simulink model "simcape_real_time_V3"  (R2022b)
settings: Solver=FixedStepAuto  StartTime=0.0  StopTime=100  FixedStep=0.002  RelTol=1e-3
undefined symbols (not defined in the file): drone_leg, K_LQR_GOC, pitch_init, roll_init, v_pitch_init, v_roll_init, v_x_init, v_y_init, v_yaw_init, v_z_init, X, x_init, Y, y_init, yaw_init, Z, z_init
libraries: sm_lib x70, nesl_utility x11, simulink x6
(part 1 of 4)
settings Model: Creator=tridu  LastModifiedBy=tridu

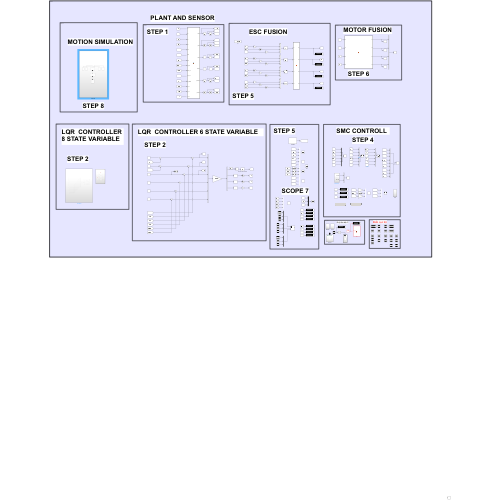
[thumbnail: Simulink's stored preview of the top-level diagram]
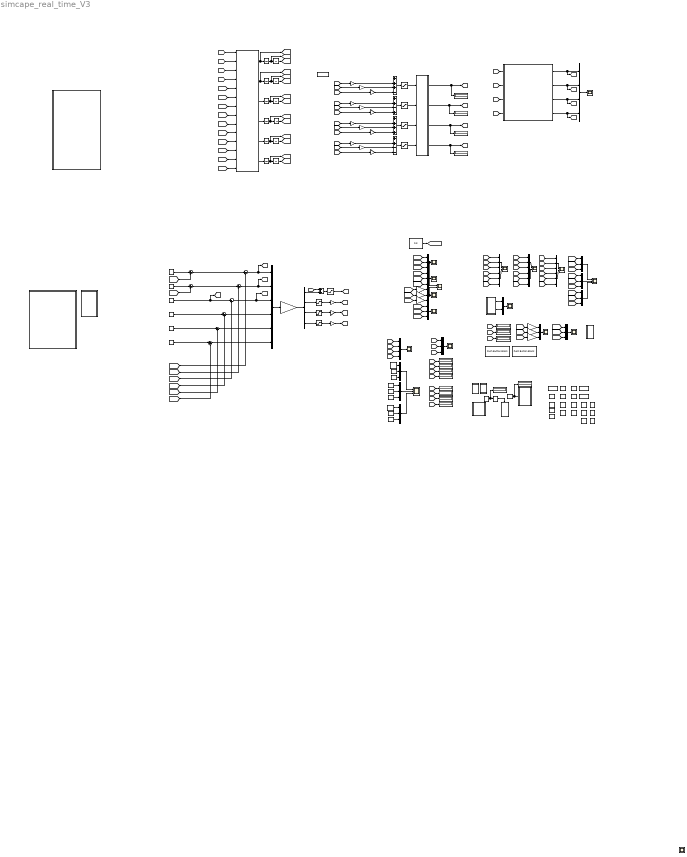
== system simcape_real_time_V3 ==
  note: STEP 2
  note: Quỹ đạo bậc 5
  note: LQR CONTROLLER 8 STATE VARIABLE
  note: Biến cục bộ
  note: Quỹ đạo
  note: STEP 5
  note: ARM 2
  note: ARM 2
  note: STEP 4
  note: ARM 2
  note: STEP 1
  note: SCOPE 7
  note: STEP 6
  note: ARM 2
  note: STEP 5
  note: SMC CONTROLL
  note: PLANT AND SENSOR
  note: LQR CONTROLLER 6 STATE VARIABLE
  note: ARM 2
  note: STEP 8
  note: MOTOR FUSION
  note: ARM 2
  note: ARM 2
  note: ARM 2
  note: ESC FUSION
  note: STEP 2
  note: MOTION SIMULATION
  Add : Sum
  Add1 : Sum  Inputs=+++-
  Add3 : Sum  Inputs=++-+
  Add4 : Sum  Inputs=++++
  Add5 : Sum  Inputs=++--
  Compare To Constant : simulink/Logic and Bit Operations/Compare To Constant  relop===  const=1  OutDataTypeStr=boolean
  Constant : Constant  Value=1.7*9.81/4
  Constant{2..3,23,25..27} (6 alike) : Constant  Value=0
  Data Store Memory : DataStoreMemory  DataStoreName=x_a  WriteAfterWriteMsg=warning  ShowAdditionalParam=off
  Data Store Memory1 : DataStoreMemory  DataStoreName=z_a  WriteAfterWriteMsg=warning  ShowAdditionalParam=off
  Data Store Memory10 : DataStoreMemory  DataStoreName=start  WriteAfterWriteMsg=warning  ShowAdditionalParam=off
  Data Store Memory11 : DataStoreMemory  DataStoreName=v_x  WriteAfterWriteMsg=warning  ShowAdditionalParam=off
  Data Store Memory12 : DataStoreMemory  DataStoreName=v_y  WriteAfterWriteMsg=warning  ShowAdditionalParam=off
  Data Store Memory13 : DataStoreMemory  DataStoreName=enable  WriteAfterWriteMsg=warning  ShowAdditionalParam=off
  Data Store Memory14 : DataStoreMemory  DataStoreName=stop  WriteAfterWriteMsg=warning  ShowAdditionalParam=off
  Data Store Memory15 : DataStoreMemory  DataStoreName=motor_13  WriteAfterWriteMsg=warning  ShowAdditionalParam=off  OutDataTypeStr=double  Dimensions=1
  Data Store Memory16 : DataStoreMemory  DataStoreName=motor_24  WriteAfterWriteMsg=warning  ShowAdditionalParam=off  OutDataTypeStr=double  Dimensions=1
  Data Store Memory17 : DataStoreMemory  DataStoreName=v_z  WriteAfterWriteMsg=warning  ShowAdditionalParam=off
  Data Store Memory18 : DataStoreMemory  DataStoreName=a_x  WriteAfterWriteMsg=warning  ShowAdditionalParam=off
  Data Store Memory19 : DataStoreMemory  DataStoreName=a_y  WriteAfterWriteMsg=warning  ShowAdditionalParam=off
  Data Store Memory2 : DataStoreMemory  DataStoreName=y_a  WriteAfterWriteMsg=warning  ShowAdditionalParam=off
  Data Store Memory20 : DataStoreMemory  DataStoreName=a_z  WriteAfterWriteMsg=warning  ShowAdditionalParam=off
  Data Store Memory3 : DataStoreMemory  DataStoreName=t  WriteAfterWriteMsg=warning  ShowAdditionalParam=off
  Data Store Memory4 : DataStoreMemory  DataStoreName=xyzv  WriteAfterWriteMsg=warning  ShowAdditionalParam=off  OutDataTypeStr=double  Dimensions=4
  Data Store Memory5 : DataStoreMemory  DataStoreName=Px_pre  WriteAfterWriteMsg=warning  ShowAdditionalParam=off
  Data Store Memory6 : DataStoreMemory  DataStoreName=Py_pre  WriteAfterWriteMsg=warning  ShowAdditionalParam=off
  Data Store Memory7 : DataStoreMemory  DataStoreName=Pz_pre  WriteAfterWriteMsg=warning  ShowAdditionalParam=off
  Data Store Memory8 : DataStoreMemory  DataStoreName=phantram_s  WriteAfterWriteMsg=warning  ShowAdditionalParam=off
  Data Store Memory9 : DataStoreMemory  DataStoreName=N_wp  WriteAfterWriteMsg=warning  ShowAdditionalParam=off
  Data Store Read : DataStoreRead  DataStoreName=v_x  IndexOptions=Index vector (dialog)  Indices=1  OutputSizes=1
  Data Store Read14 : DataStoreRead  DataStoreName=a_y  IndexOptions=Index vector (dialog)  Indices=1  OutputSizes=1
  Data Store Read15 : DataStoreRead  DataStoreName=Px_pre  IndexOptions=Index vector (dialog)  Indices=1  OutputSizes=1
  Data Store Read16 : DataStoreRead  DataStoreName=v_z  IndexOptions=Index vector (dialog)  Indices=1  OutputSizes=1
  Data Store Read17 : DataStoreRead  DataStoreName=a_z  IndexOptions=Index vector (dialog)  Indices=1  OutputSizes=1
  Data Store Read2 : DataStoreRead  DataStoreName=N_wp  DataStoreElements=N_wp  IndexOptions=Index vector (dialog)  Indices=1  OutputSizes=1
  Data Store Read3 : DataStoreRead  DataStoreName=Px_pre  IndexOptions=Index vector (dialog)  Indices=1  OutputSizes=1
  Data Store Read4 : DataStoreRead  DataStoreName=a_x  IndexOptions=Index vector (dialog)  Indices=1  OutputSizes=1
  Data Store Read7 : DataStoreRead  DataStoreName=v_y  IndexOptions=Index vector (dialog)  Indices=1  OutputSizes=1
  Data Store Read8 : DataStoreRead  DataStoreName=Pz_pre  IndexOptions=Index vector (dialog)  Indices=1  OutputSizes=1
  Data Store Read9 : DataStoreRead  DataStoreName=enable  IndexOptions=Index vector (dialog)  Indices=1  OutputSizes=1
  Demux2 : Demux
  Display{,1..12,14..17} (17 alike) : Display
  G00(xyzv) : Subsystem  TreatAsAtomicUnit=on
  Gain{8..12,14,16,18} (8 alike) : Gain  Gain=1/4
  Gain{13,15,17,19} (4 alike) : Gain  Gain=1/2
  Gain20 : Gain  Gain=0.3
  Gain24 : Gain  Gain=0.3
  Gain26 : Gain  Gain=0.1
  Gain{4..6,28..30} (6 alike) : Gain  Gain=180/pi
  Gain7 : Gain  Gain=K_LQR_GOC  Multiplication=Matrix(K*u)
  Giới hạn công suất U2 : Saturate  UpperLimit=11.5*4-1.7*9.81  LowerLimit=-1.7*9.81
  HS_MSKK : Constant  Value=0.3
  Integrator : Integrator  InitialCondition=v_x_init
  Integrator1 : Integrator  InitialCondition=x_init
  Integrator10 : Integrator  InitialCondition=v_yaw_init
  Integrator11 : Integrator  InitialCondition=yaw_init
  Integrator2 : Integrator  InitialCondition=v_y_init
  Integrator3 : Integrator  InitialCondition=y_init
  Integrator4 : Integrator  InitialCondition=z_init
  Integrator5 : Integrator  InitialCondition=v_z_init
  Integrator6 : Integrator  InitialCondition=v_roll_init
  Integrator7 : Integrator  InitialCondition=roll_init
  Integrator8 : Integrator  InitialCondition=v_pitch_init
  Integrator9 : Integrator  InitialCondition=pitch_init
  MATLAB Function : MATLAB Function  TreatAsAtomicUnit=on
  MATLAB Function1 : MATLAB Function  TreatAsAtomicUnit=on
  MATLAB Function2 : MATLAB Function  TreatAsAtomicUnit=on
  Mux{,1..3,6..9,13..23} (19 alike) : Mux  Inputs=3
  Mux10 : Mux  Inputs=6
  Mux11 : Mux
  Mux12 : Mux  Inputs=2
  Mux4 : Mux
  Nút Start : Subsystem
  Nút Stop : Subsystem
  Push Button : PushButtonBlock  ButtonText=Start  IconColor=On  OffValue=0.000000
  Push Button1 : PushButtonBlock  ButtonText=Stop  IconColor=On  OffValue=0.000000
  SIMCAPE : Subsystem
  Saturation1 : Saturate  UpperLimit=11.5  LowerLimit=-11.5
  Saturation10 : Saturate  UpperLimit=11.5  LowerLimit=-11.5
  Saturation{2..5} (4 alike) : Saturate  UpperLimit=11.5  LowerLimit=0
  Saturation8 : Saturate  UpperLimit=11.5  LowerLimit=-11.5
  Scope{,1..3,6,11..15,18} (11 alike) : Scope
  Scope16 : Scope  NumInputPorts=2
  Scope17 : Scope  NumInputPorts=3
  Scope20 : Scope  NumInputPorts=2
  Scope4 : Scope  NumInputPorts=3
  Scope9 : Scope  NumInputPorts=2
  State : Scope  NumInputPorts=2
  Subsystem : Subsystem
  Subsystem1 : Subsystem
  Subsystem3 : Subsystem
  Subsystem4 : Subsystem
  Sum : Sum  Inputs=|++
  Sum{1..4,9..10} (6 alike) : Sum  Inputs=|+-
  Sum11 : Sum  Inputs=|++
  call1 : MATLAB Function  TreatAsAtomicUnit=on
  sai số : Subsystem
  tag scope: D1=global, D2=global, D3=global, D4=global, HS_MSKK=global, T1=global, T2=global, T3=global, T4=global, U1=global, U2=global, U3=global, U4=global, e_pitch=global, e_roll=global, e_yaw=global, pitch=global, pitchdot=global, roll=global, rolldot=global, x2dot=global, x=global, xdot=global, y2dot=global, y=global, yaw=global, yaw_SP=global, yawdot=global, ydot=global, z=global, zdot=global
  wires:
  Data Store Read9/1 -> Display12/1, Compare To Constant/1
  [yaw] -> Gain30/1
  Constant27/1 -> Sum/1
  [pitch] -> MATLAB Function/6(pitch)
  Integrator1/1 -> [x]
  [U1] -> Gain12/1
  Mux15/1 -> Scope15/1
  MATLAB Function2/3(D3) -> Display2/1, [D3]
  [z] -> Mux/3
  [U4] -> Display7/1
  [yawdot] -> Mux3/3
  Gain12/1 -> Add5/2
  [pitchdot] -> Mux3/2
  Sum11/1 -> Sum10/1
  [U3] -> Mux11/3
  [U3] -> Display6/1
  [Ux] -> Mux13/1
  MATLAB Function/2(y2dot) -> [y2dot], Integrator2/1
  [pitchdot] -> MATLAB Function/9(pitch_dot)
  MATLAB Function/3(z2dot) -> Integrator4/1
  Gain13/1 -> Add3/4
  Gain11/1 -> Add3/3
  MATLAB Function1/1(T1) -> Mux4/1, [T1]
  Giới hạn công suất U2/1 -> [U1]
  [rolldot] -> Sum2/2
  Saturation3/1 -> MATLAB Function2/2(T2)
  [ydot] -> Mux1/2
  Integrator/1 -> [xdot], Integrator1/1
  Demux2/4 -> Saturation10/1
  HS_MSKK/1 -> [HS_MSKK]
  Gain5/1 -> Mux2/2
  [rolldot] -> MATLAB Function/8(roll_dot)
  Saturation5/1 -> MATLAB Function2/4(T4)
  [U4] -> Gain14/1
  Gain18/1 -> Add5/3
  Gain7/1 -> Demux2/1
  MATLAB Function2/1(D1) -> Display/1, [D1]
  [x] -> Mux/1
  Saturation10/1 -> Gain26/1
  Saturation8/1 -> Gain24/1
  Data Store Read2/1 -> Display11/1, call1/1(N_wp)
  MATLAB Function1/3(T3) -> Mux4/3, [T3]
  MATLAB Function2/4(D4) -> Display3/1, [D4]
  Gain15/1 -> Add1/4
  Integrator3/1 -> [y]
  [U2] -> Display5/1
  [U4] -> Gain18/1
  [roll] -> Gain4/1
  Sum1/1 -> [e_roll], Mux10/1
  [T1] -> MATLAB Function/1(T1)
  [x] -> Mux14/1
  Constant25/1 -> Sum3/1
  Gain29/1 -> Mux15/2
  [U2] -> Gain19/1
  Gain19/1 -> Add5/4
  [roll] -> Gain28/1
  Add4/1 -> Saturation4/1
  MATLAB Function2/2(D2) -> Display1/1, [D2]
  Demux2/2 -> Saturation1/1
  [U4] -> Gain16/1
  Demux2/3 -> Saturation8/1
  Saturation4/1 -> MATLAB Function2/3(T3)
  [U4] -> Gain11/1
  Saturation2/1 -> MATLAB Function2/1(T1)
  Mux4/1 -> Scope6/1
  [D1] -> MATLAB Function1/1(D1)
  Integrator10/1 -> [yawdot], Integrator11/1
  [zdot] -> MATLAB Function/14(z_dot)
  [y] -> Display9/1
  MATLAB Function/1(x2dot) -> [x2dot], Integrator/1
  [T2] -> MATLAB Function/2(T2)
  Gain28/1 -> Mux15/1
  [U3] -> Gain17/1
  Gain14/1 -> Add1/3
  [D2] -> MATLAB Function1/2(D2)
  MATLAB Function1/4(T4) -> Mux4/4, [T4]
  Mux12/1 -> Scope12/1
  [z] -> Display10/1
  Constant2/1 -> Sum11/1
  Add1/1 -> Saturation2/1
  [Uy] -> Mux13/2
  [U2] -> Gain13/1
  [pitch] -> Sum10/2
  Mux/1 -> State/1, Scope/1
  [y] -> Mux/2
  [yawdot] -> MATLAB Function/10(yaw_dot)
  MATLAB Function1/2(T2) -> Mux4/2, [T2]
  Integrator5/1 -> [z]
  Gain16/1 -> Add4/3
  [D4] -> MATLAB Function1/4(D4)
  Saturation1/1 -> Gain20/1
  [xdot] -> Mux1/1
  Constant26/1 -> Sum4/1
  Add3/1 -> Saturation3/1
  Sum3/1 -> Mux10/5
  Integrator2/1 -> [ydot], Integrator3/1
  [U1] -> Gain10/1
  [U2] -> Mux11/2
  Gain9/1 -> Add3/2
  [U4] -> Mux11/4
  Sum/1 -> Sum1/1
  Sum4/1 -> Mux10/6
  Subsystem4/2(Pitch SP) -> Mux12/2
  Gain8/1 -> Add1/2
  Gain4/1 -> Mux2/1
  [U1] -> Gain9/1
  Integrator6/1 -> [rolldot], Integrator7/1
  Constant23/1 -> Sum2/1
  [pitch] -> Gain5/1
  [U1] -> Gain8/1
  Gain17/1 -> Add4/4
  MATLAB Function/5(pitch2dot) -> Integrator8/1
  Sum10/1 -> [e_pitch], Mux10/2
  [U1] -> Mux11/1
  [roll_SP] -> Sum/2
  Mux13/1 -> Scope13/1
  [T1] -> Display14/1
  [xdot] -> MATLAB Function/12(x_dot)
  [x] -> Display8/1
  [T4] -> Display17/1
  [D3] -> MATLAB Function1/3(D3)
  Gain26/1 -> [U4]
  Subsystem4/1(Roll SP) -> Mux12/1
  MATLAB Function/6(yaw2dot) -> Integrator10/1
  Integrator9/1 -> [pitch]
  Integrator11/1 -> [yaw]
  [z] -> Mux14/3
  [ydot] -> MATLAB Function/13(y_dot)
  [roll] -> MATLAB Function/5(roll)
  [roll] -> Sum1/2
  Gain10/1 -> Add4/2
  Mux10/1 -> Gain7/1
  Gain6/1 -> Mux2/3
  Integrator4/1 -> [zdot], Integrator5/1
  Mux11/1 -> Scope11/1
  [rolldot] -> Mux3/1
  [T3] -> MATLAB Function/3(T3)
  Gain30/1 -> Mux15/3
  MATLAB Function/4(roll2dot) -> Integrator6/1
  Mux3/1 -> Scope3/1
  [yaw] -> Sum9/2
  [U3] -> Gain15/1
  Integrator7/1 -> [roll]
  [U1] -> Display4/1
  Mux1/1 -> Scope1/1
  Integrator8/1 -> [pitchdot], Integrator9/1
  Mux2/1 -> State/2, Scope2/1
  [HS_MSKK] -> MATLAB Function/11(HS_MSKK)
  [y] -> Mux14/2
  [yawdot] -> Sum4/2
  Mux14/1 -> Scope14/1
  Gain20/1 -> [U2]
  [T4] -> MATLAB Function/4(T4)
  [pitch_SP] -> Sum11/2
  [yaw] -> Gain6/1
  Add5/1 -> Saturation5/1
  [pitch] -> Gain29/1
  [pitchdot] -> Sum3/2
  [T3] -> Display16/1
  Gain24/1 -> [U3]
  [yaw] -> MATLAB Function/7(yaw)
  [T2] -> Display15/1
  [Uz] -> Mux13/3
  Sum2/1 -> Mux10/4
  [zdot] -> Mux1/3
  Compare To Constant/1 -> Subsystem/Enable
  Mux9/1 -> Scope17/1
  Data Store Read3/1 -> Mux9/1
  Data Store Read/1 -> Mux9/2
  Data Store Read4/1 -> Mux9/3
  Mux16/1 -> Scope17/2
  Data Store Read14/1 -> Mux16/3
  Data Store Read7/1 -> Mux16/2
  Data Store Read15/1 -> Mux16/1
  Data Store Read16/1 -> Mux17/3
  Data Store Read17/1 -> Mux17/2
  Data Store Read8/1 -> Mux17/1
  Mux17/1 -> Scope17/3
  Sum9/1 -> [e_yaw], Mux10/3
  Constant3/1 -> [yaw_SP], Sum9/1
  [roll_SP] -> Mux21/1
  [e_roll] -> Mux21/3
  [roll] -> Mux21/2
  Mux21/1 -> Scope4/1
  [pitch_SP] -> Mux6/1
  [pitch] -> Mux6/2
  [e_pitch] -> Mux6/3
  [e_yaw] -> Mux7/3
  [yaw_SP] -> Mux7/1
  [yaw] -> Mux7/2
  [x] -> Mux8/2
  Mux8/1 -> Scope9/1
  [xdot] -> Mux18/2
  Mux18/1 -> Scope9/2
  Mux19/1 -> Scope16/2
  Mux20/1 -> Scope16/1
  [y] -> Mux20/2
  [ydot] -> Mux19/2
  Mux22/1 -> Scope20/2
  Mux23/1 -> Scope20/1
  Mux6/1 -> Scope4/2
  Mux7/1 -> Scope4/3
  [z] -> Mux23/2
  [z_SP] -> Mux23/1
  [zdot] -> Mux22/2
  [zdot_SP] -> Mux22/1
  [ez] -> Mux23/3
  [ez_dot] -> Mux22/3
  [xdot_SP] -> Mux18/1
  [x_SP] -> Mux8/1
  [y_SP] -> Mux20/1
  [ydot_SP] -> Mux19/1
  [ex] -> Mux8/3
  [ex_dot] -> Mux18/3
  [ey] -> Mux20/3
  [ey_dot] -> Mux19/3
  Add/1 -> Giới hạn công suất U2/1
  [Uz] -> Add/1
  Demux2/1 -> Add/2

== system simcape_real_time_V3/G00(xyzv) ==
  MoveL : TriggerPort  TriggerType=function-call  IsSimulinkFunction=on  FunctionName=MoveL  FunctionVisibility=scoped  VariantControl=(inherit)
  Data Store Write2 : DataStoreWrite  DataStoreName=xyzv  IndexOptions=Index vector (dialog)  Indices=1  OutputSizes=1
  Display : Display
  Display1 : Display
  MATLAB Function1 : MATLAB Function  TreatAsAtomicUnit=on
  xyzv : ArgIn  DisableCoverage=on  PortDimensions=4  ArgumentName=xyzv
  wires:
  MATLAB Function1/1(xyzv_out) -> Display/1, Data Store Write2/1
  xyzv/1 -> Display1/1, MATLAB Function1/1(xyzv_in)

== system simcape_real_time_V3/Nút Start ==
  Compare To Constant10 : simulink/Logic and Bit Operations/Compare To Constant  relop===  const=1  OutDataTypeStr=boolean
  Constant : Constant
  Constant5 : Constant  Value=0
  Data Store Read1 : DataStoreRead  DataStoreName=start  DataStoreElements=start  IndexOptions=Index vector (dialog)  Indices=1  OutputSizes=1
  Data Store Write : DataStoreWrite  DataStoreName=start  IndexOptions=Index vector (dialog)  Indices=1  OutputSizes=1
  START : Subsystem  TreatAsAtomicUnit=on
  wires:
  Compare To Constant10/1 -> START/Trigger
  Constant5/1 -> Data Store Write/1
  Constant/1 -> Compare To Constant10/1

== system simcape_real_time_V3/Nút Stop ==
  Compare To Constant : simulink/Logic and Bit Operations/Compare To Constant  relop===  const=1  OutDataTypeStr=boolean
  Compare To Constant1 : simulink/Logic and Bit Operations/Compare To Constant  relop===  const=0  OutDataTypeStr=boolean
  Data Store Read : DataStoreRead  DataStoreName=stop  IndexOptions=Index vector (dialog)  Indices=1  OutputSizes=1
  Data Store Write : DataStoreWrite  DataStoreName=stop  IndexOptions=Index vector (dialog)  Indices=1  OutputSizes=1
  Stop : Constant  Value=0
  Triggered Subsystem : Subsystem  TreatAsAtomicUnit=on
  Triggered Subsystem1 : Subsystem  TreatAsAtomicUnit=on
  wires:
  Stop/1 -> Data Store Write/1
  Data Store Read/1 -> Compare To Constant/1
  Compare To Constant/1 -> Triggered Subsystem/Trigger
  [z] -> Compare To Constant1/1
  Compare To Constant1/1 -> Triggered Subsystem1/Trigger

== system simcape_real_time_V3/SIMCAPE ==
  Body : Subsystem
  MOTOR 1 : Subsystem
  MOTOR 2 : Subsystem
  MOTOR 3 : Subsystem
  MOTOR 4 : Subsystem
  Subsystem3 : Subsystem
  Subsystem5 : Subsystem
  connections:
  Subsystem3/RConn4 -- MOTOR 4/RConn1
  Subsystem5/RConn1 -- Body/LConn1
  Subsystem3/RConn3 -- MOTOR 3/LConn1
  MOTOR 2/RConn1 -- Subsystem3/RConn2
  Subsystem3/RConn1 -- MOTOR 1/LConn1
  Body/RConn1 -- Subsystem3/LConn1

== system simcape_real_time_V3/Subsystem ==
  Enable : EnablePort
  Quỹ đạo bậc 5 : Subsystem

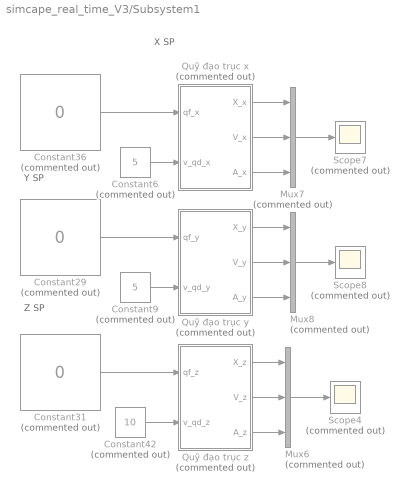
== system simcape_real_time_V3/Subsystem1 ==
  note: Z SP
  note: X SP
  note: Y SP
  Constant29 : Constant  Commented=on  Value=0
  Constant31 : Constant  Commented=on  Value=0
  Constant36 : Constant  Commented=on  Value=0
  Constant42 : Constant  Commented=on  Value=10
  Constant6 : Constant  Commented=on  Value=5
  Constant9 : Constant  Commented=on  Value=5
  Mux6 : Mux  Commented=on  Inputs=3
  Mux7 : Mux  Commented=on  Inputs=3
  Mux8 : Mux  Commented=on  Inputs=3
  Quỹ đạo trục x : Subsystem  Commented=on
  Quỹ đạo trục y : Subsystem  Commented=on
  Quỹ đạo trục z : Subsystem  Commented=on
  Scope4 : Scope  Commented=on
  Scope7 : Scope  Commented=on
  Scope8 : Scope  Commented=on
  wires:
  Constant29/1 -> Quỹ đạo trục y/1(qf_y)
  Quỹ đạo trục z/2(V_z) -> Mux6/2
  Mux6/1 -> Scope4/1
  Mux8/1 -> Scope8/1
  Quỹ đạo trục y/2(V_y) -> Mux8/2
  Constant36/1 -> Quỹ đạo trục x/1(qf_x)
  Constant42/1 -> Quỹ đạo trục z/2(v_qd_z)
  Constant6/1 -> Quỹ đạo trục x/2(v_qd_x)
  Quỹ đạo trục y/3(A_y) -> Mux8/3
  Constant9/1 -> Quỹ đạo trục y/2(v_qd_y)
  Quỹ đạo trục x/2(V_x) -> Mux7/2
  Quỹ đạo trục y/1(X_y) -> Mux8/1
  Quỹ đạo trục x/3(A_x) -> Mux7/3
  Mux7/1 -> Scope7/1
  Quỹ đạo trục z/1(X_z) -> Mux6/1
  Quỹ đạo trục x/1(X_x) -> Mux7/1
  Constant31/1 -> Quỹ đạo trục z/1(qf_z)
  Quỹ đạo trục z/3(A_z) -> Mux6/3

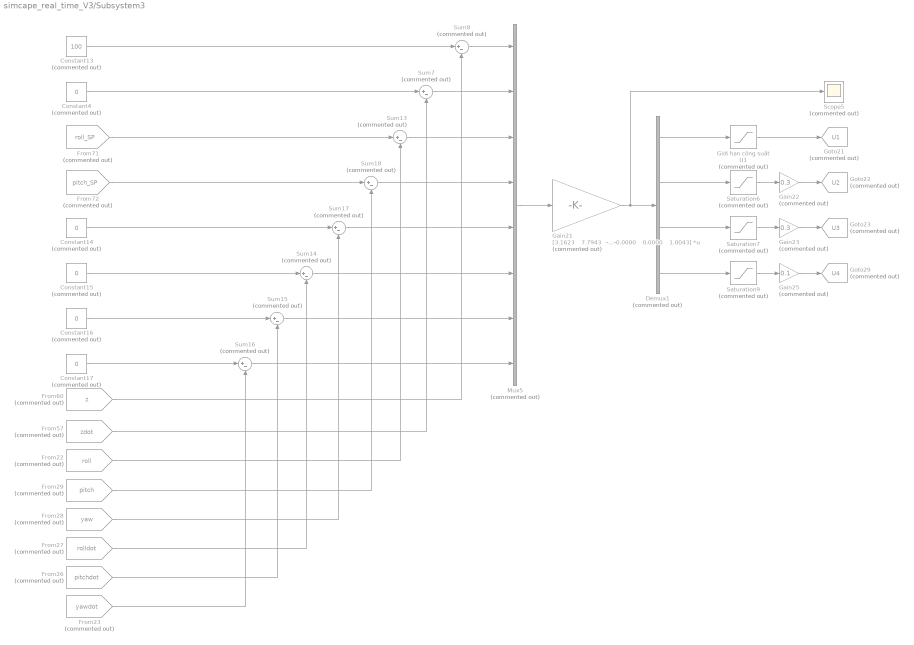
== system simcape_real_time_V3/Subsystem3 ==
  Constant13 : Constant  Commented=on  Value=100
  Constant{4,14..17} (5 alike) : Constant  Commented=on  Value=0
  Demux1 : Demux  Commented=on
  From22 : From  Commented=on  GotoTag=roll  TagVisibility=global
  From23 : From  Commented=on  GotoTag=yawdot  TagVisibility=global
  From26 : From  Commented=on  GotoTag=pitchdot  TagVisibility=global
  From27 : From  Commented=on  GotoTag=rolldot  TagVisibility=global
  From28 : From  Commented=on  GotoTag=yaw  TagVisibility=global
  From29 : From  Commented=on  GotoTag=pitch  TagVisibility=global
  From57 : From  Commented=on  GotoTag=zdot  TagVisibility=global
  From60 : From  Commented=on  GotoTag=z  TagVisibility=global
  From71 : From  Commented=on  GotoTag=roll_SP  TagVisibility=global
  From72 : From  Commented=on  GotoTag=pitch_SP  TagVisibility=global
  Gain21 : Gain  Commented=on  Gain=|  Multiplication=Matrix(K*u)
      | [3.1623    7.7943   -0.0000   -0.0000    0.0000   -0.0000   -0.0000    0.0000;
      |       -0.0000   -0.0000    3.1623   -0.0000    0.0000    1.0033   -0.0000    0.0000;
      |        0.0000   -0.0000   -0.0000    3.1623   -0.0000   -0.0000    1.0033   -0.0000;
      |        0.0000   -0.0000   -0.0000    0.0000    3.1623   -0.0000    0.0000    1.0043]
  Gain22 : Gain  Commented=on  Gain=0.3
  Gain23 : Gain  Commented=on  Gain=0.3
  Gain25 : Gain  Commented=on  Gain=0.1
  Giới hạn công suất U1 : Saturate  Commented=on  UpperLimit=29.3230*0.3  LowerLimit=-1.7*9.81
  Goto21 : Goto  Commented=on  GotoTag=U1  TagVisibility=global
  Goto22 : Goto  Commented=on  GotoTag=U2  TagVisibility=global
  Goto23 : Goto  Commented=on  GotoTag=U3  TagVisibility=global
  Goto29 : Goto  Commented=on  GotoTag=U4  TagVisibility=global
  Mux5 : Mux  Commented=on  Inputs=8
  Saturation6 : Saturate  Commented=on  UpperLimit=11.5  LowerLimit=-11.5
  Saturation7 : Saturate  Commented=on  UpperLimit=11.5  LowerLimit=-11.5
  Saturation9 : Saturate  Commented=on  UpperLimit=11.5  LowerLimit=-11.5
  Scope5 : Scope  Commented=on
  Sum{7..8,13..18} (8 alike) : Sum  Commented=on  Inputs=|+-
  wires:
  Saturation7/1 -> Gain23/1
  Sum15/1 -> Mux5/7
  From72/1 -> Sum18/1
  Sum7/1 -> Mux5/2
  Sum14/1 -> Mux5/6
  Constant14/1 -> Sum17/1
  Sum16/1 -> Mux5/8
  From29/1 -> Sum18/2
  Gain25/1 -> Goto29/1
  Constant16/1 -> Sum15/1
  Gain21/1 -> Scope5/1, Demux1/1
  Sum13/1 -> Mux5/3
  From28/1 -> Sum17/2
  Sum17/1 -> Mux5/5
  Sum18/1 -> Mux5/4
  From57/1 -> Sum7/2
  Constant4/1 -> Sum7/1
  From60/1 -> Sum8/2
  Giới hạn công suất U1/1 -> Goto21/1
  From23/1 -> Sum16/2
  Saturation6/1 -> Gain22/1
  Demux1/3 -> Saturation7/1
  From26/1 -> Sum15/2
  From27/1 -> Sum14/2
  Constant17/1 -> Sum16/1
  Gain23/1 -> Goto23/1
  Mux5/1 -> Gain21/1
  Sum8/1 -> Mux5/1
  Demux1/2 -> Saturation6/1
  Gain22/1 -> Goto22/1
  Demux1/4 -> Saturation9/1
  Demux1/1 -> Giới hạn công suất U1/1
  Saturation9/1 -> Gain25/1
  From71/1 -> Sum13/1
  Constant13/1 -> Sum8/1
  Constant15/1 -> Sum14/1
  From22/1 -> Sum13/2

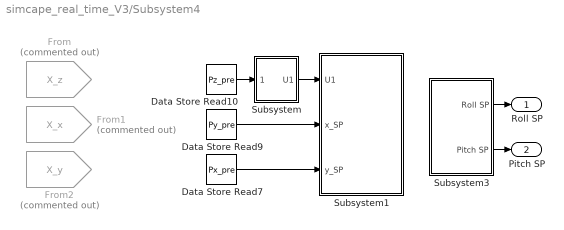
== system simcape_real_time_V3/Subsystem4 ==
  Data Store Read10 : DataStoreRead  DataStoreName=Pz_pre  IndexOptions=Index vector (dialog)  Indices=1  OutputSizes=1
  Data Store Read7 : DataStoreRead  DataStoreName=Px_pre  IndexOptions=Index vector (dialog)  Indices=1  OutputSizes=1
  Data Store Read9 : DataStoreRead  DataStoreName=Py_pre  IndexOptions=Index vector (dialog)  Indices=1  OutputSizes=1
  From : From  Commented=on  GotoTag=X_z  TagVisibility=global
  From1 : From  Commented=on  GotoTag=X_x  TagVisibility=global
  From2 : From  Commented=on  GotoTag=X_y  TagVisibility=global
  Subsystem : Subsystem
  Subsystem1 : Subsystem
  Subsystem3 : Subsystem
  Roll SP : Outport
  Pitch SP : Outport  Port=2
  wires:
  Subsystem/1(U1) -> Subsystem1/1(U1)
  Subsystem3/2(Pitch SP) -> Pitch SP/1
  Subsystem3/1(Roll SP) -> Roll SP/1
  Data Store Read7/1 -> Subsystem1/3(y_SP)
  Data Store Read10/1 -> Subsystem/1(z_SP)
  Data Store Read9/1 -> Subsystem1/2(x_SP)

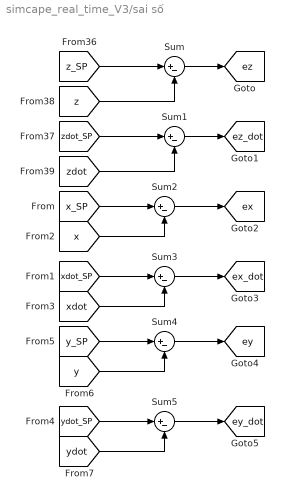
== system simcape_real_time_V3/sai số ==
  Sum{,1..5} (6 alike) : Sum  Inputs=|+-
  tag scope: ex=global, ex_dot=global, ey=global, ey_dot=global, ez=global, ez_dot=global
  wires:
  [zdot_SP] -> Sum1/1
  [z_SP] -> Sum/1
  [z] -> Sum/2
  [zdot] -> Sum1/2
  Sum/1 -> [ez]
  Sum1/1 -> [ez_dot]
  [x_SP] -> Sum2/1
  [x] -> Sum2/2
  Sum2/1 -> [ex]
  [xdot_SP] -> Sum3/1
  [xdot] -> Sum3/2
  Sum3/1 -> [ex_dot]
  [y_SP] -> Sum4/1
  [y] -> Sum4/2
  Sum4/1 -> [ey]
  [ydot_SP] -> Sum5/1
  [ydot] -> Sum5/2
  Sum5/1 -> [ey_dot]

== system simcape_real_time_V3/Nút Start/START ==
  Trigger : TriggerPort  VariantControl=Variant  InitialTriggerSignalState=zero  PortDimensions=1
  Compare To Constant : simulink/Logic and Bit Operations/Compare To Constant  relop===  const=0  OutDataTypeStr=boolean
  Constant : Constant
  Constant1 : Constant
  Constant2 : Constant  Value=-1
  Data Store Read : DataStoreRead  DataStoreName=N_wp  IndexOptions=Index vector (dialog)  Indices=1  OutputSizes=1
  Data Store Write : DataStoreWrite  DataStoreName=motor_13  IndexOptions=Index vector (dialog)  Indices=1  OutputSizes=1
  Data Store Write1 : DataStoreWrite  DataStoreName=enable  IndexOptions=Index vector (dialog)  Indices=1  OutputSizes=1
  Data Store Write2 : DataStoreWrite  DataStoreName=motor_24  IndexOptions=Index vector (dialog)  Indices=1  OutputSizes=1
  Subsystem : Subsystem
  wires:
  Compare To Constant/1 -> Subsystem/Enable
  Data Store Read/1 -> Compare To Constant/1
  Constant/1 -> Data Store Write1/1
  Constant1/1 -> Data Store Write/1
  Constant2/1 -> Data Store Write2/1

== system simcape_real_time_V3/Nút Stop/Triggered Subsystem ==
  Trigger : TriggerPort  VariantControl=(inherit)
  Constant : Constant  Value=0
  Constant1 : Constant  Value=0
  Constant2 : Constant  Value=0
  Data Store Write : DataStoreWrite  DataStoreName=enable  IndexOptions=Index vector (dialog)  Indices=1  OutputSizes=1
  Data Store Write1 : DataStoreWrite  DataStoreName=N_wp  IndexOptions=Index vector (dialog)  Indices=1  OutputSizes=1
  Data Store Write2 : DataStoreWrite  DataStoreName=Px_pre  IndexOptions=Index vector (dialog)  Indices=1  OutputSizes=1
  Data Store Write3 : DataStoreWrite  DataStoreName=Py_pre  IndexOptions=Index vector (dialog)  Indices=1  OutputSizes=1
  Data Store Write4 : DataStoreWrite  DataStoreName=Pz_pre  IndexOptions=Index vector (dialog)  Indices=1  OutputSizes=1
  wires:
  Constant/1 -> Data Store Write/1
  Constant1/1 -> Data Store Write1/1
  Constant2/1 -> Data Store Write4/1, Data Store Write3/1, Data Store Write2/1

== system simcape_real_time_V3/Nút Stop/Triggered Subsystem1 ==
  Trigger : TriggerPort  VariantControl=(inherit)
  Constant : Constant  Value=0
  Data Store Write : DataStoreWrite  DataStoreName=motor_13  IndexOptions=Index vector (dialog)  Indices=1  OutputSizes=1
  Data Store Write1 : DataStoreWrite  DataStoreName=motor_24  IndexOptions=Index vector (dialog)  Indices=1  OutputSizes=1
  wires:
  Constant/1 -> Data Store Write1/1, Data Store Write/1

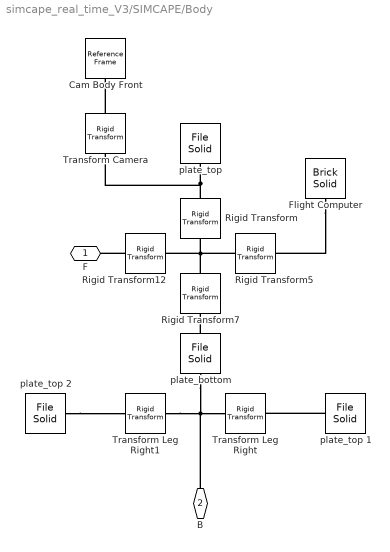
== system simcape_real_time_V3/SIMCAPE/Body ==
  Cam Body Front : sm_lib/Frames and Transforms/Reference Frame
  Flight Computer : sm_lib/Body Elements/Brick Solid  GraphicAmbientColor=[0.15 0.15 0.15 1.0]  BasedOnType=Mass  BrickDimensions=3*[20 20 5]  BrickDimensionUnits=mm  CenterOfMass=[0 0 0]  CenterOfMassUnits=m  GraphicDiffuseColor=[0.5 0.5 0.5]  Density=1000  DensityUnits=kg/m^3  DoExposeReferenceFrame=on  GraphicEmissiveColor=[0.0 0.0 0.0 1.0]  ExportEntireGeometry=off  SerializedFrames=<Frames/>  MarkerShape=Sphere  MarkerSize=10  GraphicType=FromGeometry  InertiaType=CalculateFromGeometry  Mass=638  MassUnits=g  MomentsOfInertia=[1 1 1]  MomentsOfInertiaUnits=kg*m^2  GraphicOpacity=1.0  ProductsOfInertia=[0 0 0]  ProductsOfInertiaUnits=kg*m^2  GraphicShininess=75  GraphicSpecularColor=[0.5 0.5 0.5 1.0]  GraphicVisPropType=SimpleVisualProperties
  Rigid Transform : sm_lib/Frames and Transforms/Rigid Transform  TranslationMethod=None  TranslationStandardOffset=0  TranslationLengthUnit=m  TranslationStandardAxis=+Z  TranslationCartesianOffset=[0 0 0]  TranslationROffset=0  TranslationROffsetUnits=m  TranslationZOffset=0  TranslationZOffsetUnits=m  TranslationThetaOffset=0  TranslationThetaOffsetUnits=deg  RotationMethod=None  RotationAngleUnits=deg  RotationStandardAxis=+Z  RotationAngle=45  RotationArbitraryAxis=[0 0 1]  FollAlignAxisA=+X  BaseAlignAxisA=+Y  FollAlignAxisB=+Y  BaseAlignAxisB=+Z  RotationSequenceAxes=FollowerAxes  RotationSequence=XYX  RotationSequenceAngles=[0 0 0]  RotationSequenceAnglesUnits=deg  RotationMatrix=[1 0 0; 0 1 0; 0 0 1]  Quaternion=[1 0 0 0]
  Rigid Transform12 : sm_lib/Frames and Transforms/Rigid Transform  TranslationMethod=Cartesian  TranslationStandardOffset=0  TranslationLengthUnit=mm  TranslationStandardAxis=+Z  TranslationCartesianOffset=[0 0 -26]  TranslationROffset=0  TranslationROffsetUnits=m  TranslationZOffset=0  TranslationZOffsetUnits=m  TranslationThetaOffset=0  TranslationThetaOffsetUnits=deg  RotationMethod=None  RotationAngleUnits=deg  RotationStandardAxis=+Z  RotationAngle=45  RotationArbitraryAxis=[0 0 1]  FollAlignAxisA=+X  BaseAlignAxisA=+Y  FollAlignAxisB=+Y  BaseAlignAxisB=+Z  RotationSequenceAxes=FollowerAxes  RotationSequence=XYX  RotationSequenceAngles=[0 0 0]  RotationSequenceAnglesUnits=deg  RotationMatrix=[1 0 0; 0 1 0; 0 0 1]  Quaternion=[1 0 0 0]
  Rigid Transform5 : sm_lib/Frames and Transforms/Rigid Transform  TranslationMethod=Cartesian  TranslationStandardOffset=0  TranslationLengthUnit=mm  TranslationStandardAxis=+Z  TranslationCartesianOffset=[0 0 -26]  TranslationROffset=0  TranslationROffsetUnits=m  TranslationZOffset=0  TranslationZOffsetUnits=m  TranslationThetaOffset=0  TranslationThetaOffsetUnits=deg  RotationMethod=None  RotationAngleUnits=deg  RotationStandardAxis=+Z  RotationAngle=45  RotationArbitraryAxis=[0 0 1]  FollAlignAxisA=+X  BaseAlignAxisA=+Y  FollAlignAxisB=+Y  BaseAlignAxisB=+Z  RotationSequenceAxes=FollowerAxes  RotationSequence=XYX  RotationSequenceAngles=[0 0 0]  RotationSequenceAnglesUnits=deg  RotationMatrix=[1 0 0; 0 1 0; 0 0 1]  Quaternion=[1 0 0 0]
  Rigid Transform7 : sm_lib/Frames and Transforms/Rigid Transform  TranslationMethod=Cartesian  TranslationStandardOffset=0  TranslationLengthUnit=mm  TranslationStandardAxis=+Z  TranslationCartesianOffset=[0 0 -38]  TranslationROffset=0  TranslationROffsetUnits=m  TranslationZOffset=0  TranslationZOffsetUnits=m  TranslationThetaOffset=0  TranslationThetaOffsetUnits=deg  RotationMethod=None  RotationAngleUnits=deg  RotationStandardAxis=+Z  RotationAngle=45  RotationArbitraryAxis=[0 0 1]  FollAlignAxisA=+X  BaseAlignAxisA=+Y  FollAlignAxisB=+Y  BaseAlignAxisB=+Z  RotationSequenceAxes=FollowerAxes  RotationSequence=XYX  RotationSequenceAngles=[0 0 0]  RotationSequenceAnglesUnits=deg  RotationMatrix=[1 0 0; 0 1 0; 0 0 1]  Quaternion=[1 0 0 0]
  Transform Camera : sm_lib/Frames and Transforms/Rigid Transform  TranslationMethod=Cartesian  TranslationStandardOffset=0  TranslationLengthUnit=m  TranslationStandardAxis=+Z  TranslationCartesianOffset=[0.06 0 0]  TranslationROffset=0  TranslationROffsetUnits=m  TranslationZOffset=0  TranslationZOffsetUnits=m  TranslationThetaOffset=0  TranslationThetaOffsetUnits=deg  RotationMethod=None  RotationAngleUnits=deg  RotationStandardAxis=+Z  RotationAngle=0.0  RotationArbitraryAxis=[0 0 1]  FollAlignAxisA=+X  BaseAlignAxisA=+Y  FollAlignAxisB=+Y  BaseAlignAxisB=+Z  RotationSequenceAxes=FollowerAxes  RotationSequence=XYX  RotationSequenceAngles=[0 0 0]  RotationSequenceAnglesUnits=deg  RotationMatrix=[1 0 0; 0 1 0; 0 0 1]  Quaternion=[1 0 0 0]
  Transform Leg Right : sm_lib/Frames and Transforms/Rigid Transform  TranslationMethod=Cartesian  TranslationStandardOffset=0.09-drone_leg.width/2  TranslationLengthUnit=m  TranslationStandardAxis=-Y  TranslationCartesianOffset=[0 -0.08 -0.001]  TranslationROffset=0  TranslationROffsetUnits=m  TranslationZOffset=0  TranslationZOffsetUnits=m  TranslationThetaOffset=0  TranslationThetaOffsetUnits=deg  RotationMethod=StandardAxis  RotationAngleUnits=deg  RotationStandardAxis=-X  RotationAngle=180  RotationArbitraryAxis=[0 0 1]  FollAlignAxisA=+X  BaseAlignAxisA=+Y  FollAlignAxisB=+Y  BaseAlignAxisB=+Z  RotationSequenceAxes=FollowerAxes  RotationSequence=XYX  RotationSequenceAngles=[0 0 0]  RotationSequenceAnglesUnits=deg  RotationMatrix=[1 0 0; 0 1 0; 0 0 1]  Quaternion=[1 0 0 0]
  Transform Leg Right1 : sm_lib/Frames and Transforms/Rigid Transform  TranslationMethod=Cartesian  TranslationStandardOffset=0.09-drone_leg.width/2  TranslationLengthUnit=m  TranslationStandardAxis=-Y  TranslationCartesianOffset=[0 0.08 -0.001]  TranslationROffset=0  TranslationROffsetUnits=m  TranslationZOffset=0  TranslationZOffsetUnits=m  TranslationThetaOffset=0  TranslationThetaOffsetUnits=deg  RotationMethod=StandardAxis  RotationAngleUnits=deg  RotationStandardAxis=-X  RotationAngle=180  RotationArbitraryAxis=[0 0 1]  FollAlignAxisA=+X  BaseAlignAxisA=+Y  FollAlignAxisB=+Y  BaseAlignAxisB=+Z  RotationSequenceAxes=FollowerAxes  RotationSequence=XYX  RotationSequenceAngles=[0 0 0]  RotationSequenceAnglesUnits=deg  RotationMatrix=[1 0 0; 0 1 0; 0 0 1]  Quaternion=[1 0 0 0]
  plate_bottom : sm_lib/Body Elements/File Solid  ExtGeomFileName=C:\Users\tridu\OneDrive\Máy tính\(1)\mohinh\quadcopter_simscape\Quadcopter-Simulation-master\Quadcopter-Simulation-master\CAD\Geometry\quadcopter_drone_plate_bottom.stp  UnitType=FromFile  ExtGeomFileUnits=m  StepReaderType=HEX  ExportConvexHullGeometry=off  InertiaType=Custom  Mass=0.0317292  MassUnits=kg  CenterOfMass=[9.57262e-08, 1.0716e-07, -1.47882e-10]  CenterOfMassUnits=m  MomentsOfInertia=[2.77785e-05, 2.75764e-05, 5.53432e-05]  MomentsOfInertiaUnits=kg*m^2  ProductsOfInertia=[-9.24719e-13, -9.71809e-13, 1.0181e-10]  ProductsOfInertiaUnits=kg*m^2  BasedOnType=Density  Density=1  DensityUnits=g/cm^3  DoExposeReferenceFrame=off  SerializedFrames=<Frames><Frame><Id>Frame1</Id><Value><Name>Bot</Name><Origin><Source>GeometricFeature</Source><FeatureName>planar surface 33</FeatureName></Origin><PrimaryAxis><DefinedDirection>+Z</DefinedDirection><Source>ReferenceFrame</Source><SourceDirection>+Z</SourceDirection><FeatureName></FeatureName></PrimaryAxis><SecondaryAxis><DefinedDirection>+X</DefinedDirection><Source>ReferenceFrame</Source><SourceDirection>+Y</SourceDirection><FeatureName></FeatureName></SecondaryAxis></Value></Frame><Frame><Id>Frame2</Id><Value><Name>Top</Name><Origin><Source>ReferenceFrame</Source><FeatureName></FeatureName></Origin><PrimaryAxis><DefinedDirection>+Z</DefinedDirection><Source>ReferenceFrame</Source><SourceDirection>+Z</SourceDirection><FeatureName></FeatureName></PrimaryAxis><SecondaryAxis><DefinedDirection>+X</DefinedDirection><Source>ReferenceFrame</Source><SourceDirection>+Y</SourceDirection><FeatureName></FeatureName></SecondaryAxis></Value></Frame></Frames>  GraphicType=FromGeometry  MarkerShape=Sphere  MarkerSize=10  GraphicVisPropType=SimpleVisualProperties  GraphicDiffuseColor=[0.0 0.0 0.0]  GraphicSpecularColor=[0.5 0.5 0.5 1.0]  GraphicAmbientColor=[0.15 0.15 0.15 1.0]  GraphicEmissiveColor=[0.0 0.0 0.0 1.0]  GraphicShininess=75  GraphicOpacity=1.0
  "plate_top " : sm_lib/Body Elements/File Solid  ExtGeomFileName=C:\Users\tridu\OneDrive\Máy tính\(1)\mohinh\quadcopter_simscape\Quadcopter-Simulation-master\Quadcopter-Simulation-master\CAD\Geometry\quadcopter_drone_plate_top.stp  UnitType=FromFile  ExtGeomFileUnits=m  StepReaderType=HEX  ExportConvexHullGeometry=off  InertiaType=Custom  Mass=0.0317292  MassUnits=kg  CenterOfMass=[9.57262e-08, 1.0716e-07, -1.47882e-10]  CenterOfMassUnits=m  MomentsOfInertia=[2.77785e-05, 2.75764e-05, 5.53432e-05]  MomentsOfInertiaUnits=kg*m^2  ProductsOfInertia=[-9.24719e-13, -9.71809e-13, 1.0181e-10]  ProductsOfInertiaUnits=kg*m^2  BasedOnType=Density  Density=1  DensityUnits=g/cm^3  DoExposeReferenceFrame=on  SerializedFrames=<Frames/>  GraphicType=FromGeometry  MarkerShape=Sphere  MarkerSize=10  GraphicVisPropType=SimpleVisualProperties  GraphicDiffuseColor=[0.0 0.0 0.0]  GraphicSpecularColor=[0.5 0.5 0.5 1.0]  GraphicAmbientColor=[0.15 0.15 0.15 1.0]  GraphicEmissiveColor=[0.0 0.0 0.0 1.0]  GraphicShininess=75  GraphicOpacity=1.0
  plate_top 1 : sm_lib/Body Elements/File Solid  ExtGeomFileName=C:\Users\tridu\OneDrive\Máy tính\Code Matlad\CODE_SMC\simcape_smc_real_time\CAD\Geometry\cangv2.STEP  UnitType=FromFile  ExtGeomFileUnits=m  StepReaderType=HEX  ExportConvexHullGeometry=off  InertiaType=Custom  Mass=0.0317292  MassUnits=kg  CenterOfMass=[9.57262e-08, 1.0716e-07, -1.47882e-10]  CenterOfMassUnits=m  MomentsOfInertia=[2.77785e-05, 2.75764e-05, 5.53432e-05]  MomentsOfInertiaUnits=kg*m^2  ProductsOfInertia=[-9.24719e-13, -9.71809e-13, 1.0181e-10]  ProductsOfInertiaUnits=kg*m^2  BasedOnType=Density  Density=1  DensityUnits=g/cm^3  DoExposeReferenceFrame=on  SerializedFrames=<Frames/>  GraphicType=FromGeometry  MarkerShape=Sphere  MarkerSize=10  GraphicVisPropType=FromFileVisualProperties  GraphicDiffuseColor=[0.0 0.0 0.0]  GraphicSpecularColor=[0.5 0.5 0.5 1.0]  GraphicAmbientColor=[0.15 0.15 0.15 1.0]  GraphicEmissiveColor=[0.0 0.0 0.0 1.0]  GraphicShininess=75  GraphicOpacity=1.0
  plate_top 2 : sm_lib/Body Elements/File Solid  ExtGeomFileName=C:\Users\tridu\OneDrive\Máy tính\Code Matlad\CODE_SMC\simcape_smc_real_time\CAD\Geometry\cangv2.STEP  UnitType=FromFile  ExtGeomFileUnits=m  StepReaderType=HEX  ExportConvexHullGeometry=off  InertiaType=Custom  Mass=0.0317292  MassUnits=kg  CenterOfMass=[9.57262e-08, 1.0716e-07, -1.47882e-10]  CenterOfMassUnits=m  MomentsOfInertia=[2.77785e-05, 2.75764e-05, 5.53432e-05]  MomentsOfInertiaUnits=kg*m^2  ProductsOfInertia=[-9.24719e-13, -9.71809e-13, 1.0181e-10]  ProductsOfInertiaUnits=kg*m^2  BasedOnType=Density  Density=1  DensityUnits=g/cm^3  DoExposeReferenceFrame=on  SerializedFrames=<Frames/>  GraphicType=FromGeometry  MarkerShape=Sphere  MarkerSize=10  GraphicVisPropType=FromFileVisualProperties  GraphicDiffuseColor=[0.0 0.0 0.0]  GraphicSpecularColor=[0.5 0.5 0.5 1.0]  GraphicAmbientColor=[0.15 0.15 0.15 1.0]  GraphicEmissiveColor=[0.0 0.0 0.0 1.0]  GraphicShininess=75  GraphicOpacity=1.0
  F : PMIOPort  Side=Right
  B : PMIOPort  Port=2  Side=Left
  connections:
  Flight Computer/RConn1 -- Rigid Transform5/RConn1
  Rigid Transform7/LConn1 -- Rigid Transform5/LConn1 -- Rigid Transform12/LConn1 -- Rigid Transform/LConn1
  plate_bottom/RConn1 -- Rigid Transform7/RConn1
  Rigid Transform12/RConn1 -- F/RConn1
  Rigid Transform/RConn1 -- Transform Camera/LConn1 -- "plate_top "/RConn1
  Transform Camera/RConn1 -- Cam Body Front/RConn1
  plate_top 1/RConn1 -- Transform Leg Right/RConn1
  Transform Leg Right1/LConn1 -- B/RConn1 -- plate_bottom/LConn1 -- Transform Leg Right/LConn1
  plate_top 2/RConn1 -- Transform Leg Right1/RConn1

== system simcape_real_time_V3/SIMCAPE/MOTOR 1 ==
  note: ARM 2
  note: MOTOR 1
  Cap1 : sm_lib/Body Elements/File Solid  ExtGeomFileName=C:\Users\tridu\OneDrive\Máy tính\Code Matlad\CODE_SMC\simcape_smc_real_time\CAD\Geometry\quadcopter_drone_motor_cap.stp  UnitType=FromFile  ExtGeomFileUnits=m  StepReaderType=HEX  ExportConvexHullGeometry=off  InertiaType=Custom  Mass=0.000930841  MassUnits=kg  CenterOfMass=[0 0.00200877 0]  CenterOfMassUnits=m  MomentsOfInertia=[1.32154e-08, 2.22535e-08, 1.32154e-08]  MomentsOfInertiaUnits=kg*m^2  ProductsOfInertia=[0 0 0]  ProductsOfInertiaUnits=kg*m^2  BasedOnType=Density  Density=1  DensityUnits=g/cm^3  DoExposeReferenceFrame=on  SerializedFrames=<Frames/>  GraphicType=FromGeometry  MarkerShape=Sphere  MarkerSize=10  GraphicVisPropType=AdvancedVisualProperties  GraphicDiffuseColor=[0.05 0.05 0.05]  GraphicSpecularColor=[0.5 0.5 0.5 1.0]  GraphicAmbientColor=[0.15 0.15 0.15 1.0]  GraphicEmissiveColor=[0.0 0.0 0.0 1.0]  GraphicShininess=40  GraphicOpacity=1.0
  Data Store Read10 : DataStoreRead  DataStoreName=motor_13  IndexOptions=Index vector (dialog)  Indices=1  OutputSizes=1
  Housing1 : sm_lib/Body Elements/File Solid  ExtGeomFileName=C:\Users\tridu\OneDrive\Máy tính\Code Matlad\CODE_SMC\simcape_smc_real_time\CAD\Geometry\quadcopter_drone_motor.stp  UnitType=FromFile  ExtGeomFileUnits=m  StepReaderType=HEX  ExportConvexHullGeometry=off  InertiaType=Custom  Mass=51  MassUnits=g  CenterOfMass=[0, 0, -0.0088876]  CenterOfMassUnits=m  MomentsOfInertia=[7.0438e-06, 7.04379e-06, 6.06908e-06]  MomentsOfInertiaUnits=kg*m^2  ProductsOfInertia=[0 0 0]  ProductsOfInertiaUnits=kg*m^2  BasedOnType=Mass  Density=1000  DensityUnits=kg/m^3  DoExposeReferenceFrame=on  SerializedFrames=<Frames><Frame><Id>Frame1</Id><Value><Name>F1</Name><Origin><Source>CenterOfMassFrame</Source><FeatureName></FeatureName></Origin><PrimaryAxis><DefinedDirection>-Z</DefinedDirection><Source>ReferenceFrame</Source><SourceDirection>+Z</SourceDirection><FeatureName></FeatureName></PrimaryAxis><SecondaryAxis><DefinedDirection>+X</DefinedDirection><Source>ReferenceFrame</Source><SourceDirection>+X</SourceDirection><FeatureName></FeatureName></SecondaryAxis></Value></Frame></Frames>  GraphicType=FromGeometry  MarkerShape=Sphere  MarkerSize=10  GraphicVisPropType=SimpleVisualProperties  GraphicDiffuseColor=[0.6 0.0 0.2]  GraphicSpecularColor=[0.5 0.5 0.5 1.0]  GraphicAmbientColor=[0.15 0.15 0.15 1.0]  GraphicEmissiveColor=[0.0 0.0 0.0 1.0]  GraphicShininess=75  GraphicOpacity=1.0
  Propeller1 : sm_lib/Body Elements/File Solid  ExtGeomFileName=C:\Users\tridu\OneDrive\Máy tính\Code Matlad\CODE_LQR\simcape_real_time\CAD\Geometry\quadcopter_drone_propeller_1_4.stp  UnitType=FromFile  ExtGeomFileUnits=m  StepReaderType=HEX  ExportConvexHullGeometry=off  InertiaType=Custom  Mass=0.0249468  MassUnits=kg  CenterOfMass="[0  0.00566766 0]"  CenterOfMassUnits=m  MomentsOfInertia=[0.000160013, 0.000160582, 8.20018e-07]  MomentsOfInertiaUnits=kg*m^2  ProductsOfInertia=[0 0 0]  ProductsOfInertiaUnits=kg*m^2  BasedOnType=Density  Density=1  DensityUnits=g/cm^3  DoExposeReferenceFrame=on  SerializedFrames=<Frames><Frame><Id>Frame1</Id><Value><Name>R2</Name><Origin><Source>ReferenceFrame</Source><FeatureName></FeatureName></Origin><PrimaryAxis><DefinedDirection>+Z</DefinedDirection><Source>ReferenceFrame</Source><SourceDirection>+Z</SourceDirection><FeatureName></FeatureName></PrimaryAxis><SecondaryAxis><DefinedDirection>+X</DefinedDirection><Source>ReferenceFrame</Source><SourceDirection>+X</SourceDirection><FeatureName></FeatureName></SecondaryAxis></Value></Frame></Frames>  GraphicType=FromGeometry  MarkerShape=Sphere  MarkerSize=10  GraphicVisPropType=AdvancedVisualProperties  GraphicDiffuseColor=[0.05 0.05 0.05]  GraphicSpecularColor=[0.5 0.5 0.5 1.0]  GraphicAmbientColor=[0.15 0.15 0.15 1.0]  GraphicEmissiveColor=[0.0 0.0 0.0 1.0]  GraphicShininess=40  GraphicOpacity=1.0
  Revolute Joint3 : sm_lib/Joints/Revolute Joint  JointMode=Normal  SenseConstraintForce=off  SenseConstraintForceX=off  SenseConstraintForceY=off  SenseConstraintForceZ=off  SenseConstraintTorque=off  SenseConstraintTorqueX=off  SenseConstraintTorqueY=off  SenseConstraintTorqueZ=off  SenseTotalForce=off  SenseTotalForceX=off  SenseTotalForceY=off  SenseTotalForceZ=off  SenseTotalTorque=off  SenseTotalTorqueX=off  SenseTotalTorqueY=off  SenseTotalTorqueZ=off  CompositeWrenchDir=FollowerOnBase  CompositeWrenchFrame=BaseFrame  EquilibriumPosition=0  EquilibriumPositionUnits=deg  SpringStiffness=0  SpringStiffnessUnits=N*m/rad  DampingCoefficient=1e-5  DampingCoefficientUnits=N*m/(rad/s)  TorqueActuationMode=InputTorque  MotionActuationMode=ComputedMotion  SensePosition=off  SenseVelocity=on  SenseAcceleration=off  SenseTorqueForce=off  SenseLowerLimitTorqueForce=off  SenseUpperLimitTorqueForce=off  LowerLimitSpecify=off  LowerLimitBound=-90  LowerLimitBoundUnits=deg  LowerLimitStiffness=1e4  LowerLimitStiffnessUnits=N*m/deg  LowerLimitDamping=10  LowerLimitDampingUnits=N*m/(deg/s)  LowerLimitTransitionRegionWidth=0.1  LowerLimitTransitionRegionWidthUnits=deg  UpperLimitSpecify=off  UpperLimitBound=90  UpperLimitBoundUnits=deg  UpperLimitStiffness=1e4  UpperLimitStiffnessUnits=N*m/deg  UpperLimitDamping=10  UpperLimitDampingUnits=N*m/(deg/s)  UpperLimitTransitionRegionWidth=0.1  UpperLimitTransitionRegionWidthUnits=deg  PositionTargetSpecify=off  PositionTargetPriority=High  PositionTargetValue=0  PositionTargetValueUnits=deg  VelocityTargetSpecify=off  VelocityTargetPriority=High  VelocityTargetValue=0  VelocityTargetValueUnits=deg/s
  Rigid Transform5 : sm_lib/Frames and Transforms/Rigid Transform  TranslationMethod=Cartesian  TranslationStandardOffset=90  TranslationLengthUnit=cm  TranslationStandardAxis=-Y  TranslationCartesianOffset=[0 1.5 0]  TranslationROffset=0  TranslationROffsetUnits=m  TranslationZOffset=0  TranslationZOffsetUnits=m  TranslationThetaOffset=90  TranslationThetaOffsetUnits=deg  RotationMethod=StandardAxis  RotationAngleUnits=deg  RotationStandardAxis=-X  RotationAngle=90  RotationArbitraryAxis=[0 0 1]  FollAlignAxisA=+X  BaseAlignAxisA=+Y  FollAlignAxisB=+Y  BaseAlignAxisB=+Z  RotationSequenceAxes=FollowerAxes  RotationSequence=XYX  RotationSequenceAngles=[0 0 0]  RotationSequenceAnglesUnits=deg  RotationMatrix=[1 0 0; 0 1 0; 0 0 1]  Quaternion=[1 0 0 0]
  Simulink-PS Converter2 : nesl_utility/Simulink-PS Converter  PhysicalDomain=network_engine_domain  SubClassName=ps_input  LeftPortType=input  RightPortType=output  PseudoPeriodic=off  Frequencies=[]  NoiseDistribution=none  NoiseParameters=[]  Unit=1  AffineConversion=off  FilteringAndDerivatives=zero  SimscapeFilterOrder=1  InputFilterTimeConstant=0.001  UdotUserProvided=1
  Transform Propeller1 : sm_lib/Frames and Transforms/Rigid Transform  TranslationMethod=Cartesian  TranslationStandardOffset=0  TranslationLengthUnit=mm  TranslationStandardAxis=+Z  TranslationCartesianOffset=[0 0 -20]  TranslationROffset=0  TranslationROffsetUnits=m  TranslationZOffset=0  TranslationZOffsetUnits=m  TranslationThetaOffset=0  TranslationThetaOffsetUnits=deg  RotationMethod=StandardAxis  RotationAngleUnits=deg  RotationStandardAxis=-X  RotationAngle=90  RotationArbitraryAxis=[0 0 1]  FollAlignAxisA=+X  BaseAlignAxisA=+Y  FollAlignAxisB=+Y  BaseAlignAxisB=+Z  RotationSequenceAxes=FollowerAxes  RotationSequence=XYX  RotationSequenceAngles=[0 0 0]  RotationSequenceAnglesUnits=deg  RotationMatrix=[1 0 0; 0 1 0; 0 0 1]  Quaternion=[1 0 0 0]
  Transform1 : sm_lib/Frames and Transforms/Rigid Transform  TranslationMethod=StandardAxis  TranslationStandardOffset=0.0097  TranslationLengthUnit=m  TranslationStandardAxis=+Y  TranslationCartesianOffset=[0 0 5]  TranslationROffset=0  TranslationROffsetUnits=m  TranslationZOffset=0  TranslationZOffsetUnits=m  TranslationThetaOffset=0  TranslationThetaOffsetUnits=deg  RotationMethod=None  RotationAngleUnits=deg  RotationStandardAxis=+X  RotationAngle=-90  RotationArbitraryAxis=[0 0 1]  FollAlignAxisA=+X  BaseAlignAxisA=+Y  FollAlignAxisB=+Y  BaseAlignAxisB=+Z  RotationSequenceAxes=FollowerAxes  RotationSequence=XYX  RotationSequenceAngles=[0 0 0]  RotationSequenceAnglesUnits=deg  RotationMatrix=[1 0 0; 0 1 0; 0 0 1]  Quaternion=[1 0 0 0]
  Conn1 : PMIOPort  Side=Left
  wires:
  Data Store Read10/1 -> Simulink-PS Converter2/1
  connections:
  Cap1/RConn1 -- Transform1/RConn1
  Simulink-PS Converter2/RConn1 -- Revolute Joint3/LConn2
  Housing1/LConn1 -- Revolute Joint3/RConn1
  Transform1/LConn1 -- Propeller1/LConn1
  Revolute Joint3/LConn1 -- Rigid Transform5/RConn1
  Propeller1/RConn1 -- Transform Propeller1/RConn1
  Transform Propeller1/LConn1 -- Housing1/RConn1
  Conn1/RConn1 -- Rigid Transform5/LConn1
